simulink library "wind_gust_lib"  (R2015a)
settings: Solver=ode45  SolverMode=SingleTasking  StartTime=0.0  StopTime=10.0  RelTol=1e-3
undefined symbols (not defined in the file): a, b, Mq, Mw, Swg, Vto, Zw
libraries: simulink x1
settings Model: FPTRunName=Active  ModifiedByFormat=The MathWorks Inc.  CovSFcnEnable=off  ExtModeAutoUpdateStatusClock=off  Creator=The MathWorks Inc.  LastModifiedBy=The MathWorks Inc.
settings ConfigSet: ConfigType=Model
settings SolverCC: Priority=auto
settings DataIOCC: SignalLoggingSaveFormat=ModelDataLogs
settings OptimizationCC: BlockReduction=off  BooleanDataType=off  InlineParamsCompatibleMode=off  ExpressionDepthLimit=2147483647  ForceBlockIOInitOptimize=off  EvaledLifeSpan=1  SimCompilerOptimization=Off
settings DebuggingCC: SaveWithParameterizedLinksMsg=none  UnderspecifiedInitializationDetection=Classic  MergeDetectMultiDrivingBlocksExec=none  SignalResolutionControl=TryResolveAllWithWarning  FcnCallInpInsideContextMsg=EnableAllAsWarning  AllowSymbolicDim=off  StateNameClashWarn=warning  StrictBusMsg=Warning  SFMismatchInSimAndRtwBecauseOfMissingDataTypeDiag=warning
settings HardwareCC: TargetUnknown=on
settings RTWCC: EnableTagging=off  RTWCompilerOptimization=Off
settings CodeAppCC: ParameterTuningSideEffectCode=Output function  AllmanStyle=off
settings GRTTargetCC: CombineOutputUpdateFcns=off  EnableShiftOperators=off  PortableWordSizesTransition=off  GenerateErtSFunctionTransition=off  CreateSILPILBlockTransition=None  CodeProfilingSaveOptionsTransition=SummaryOnly  CodeExecutionProfilingTransition=off  CodeProfilingInstrumentationTransition=off  CodeExecutionProfileVariableTransition=executionProfile  GRTInterface=on

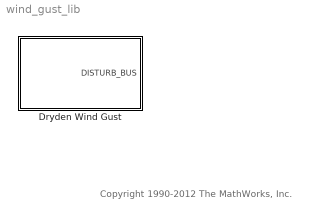
== system wind_gust_lib ==
  note: Copyright 1990-2012 The MathWorks, Inc.
  Dryden Wind Gust : Subsystem  IOType=none  Commented=off  StatePerturbationForJacobian=1.0e-05

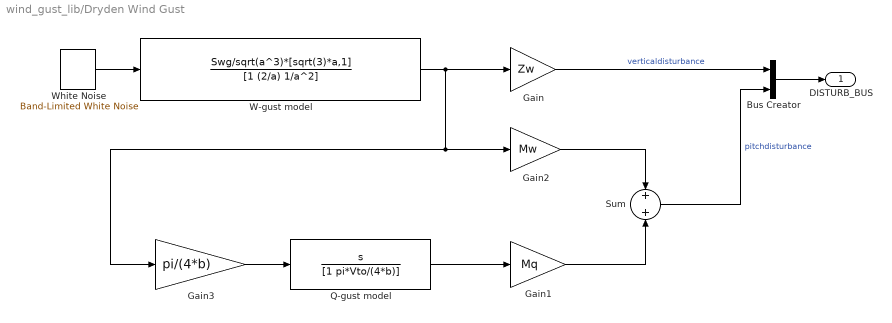
== system wind_gust_lib/Dryden Wind Gust ==
  Bus Creator : BusCreator  IOType=none  Commented=off  StatePerturbationForJacobian=1.0e-05  Inputs='verticaldisturbance','pitchdisturbance'  OutDataTypeStr=Bus: DISTURB_BUS
  Gain : Gain  IOType=none  Commented=off  StatePerturbationForJacobian=1.0e-05  Gain=Zw  SaturateOnIntegerOverflow=on  OutDataTypeStr=Inherit: Same as input  ParamDataTypeStr=Inherit: Same as input
  Gain1 : Gain  IOType=none  Commented=off  StatePerturbationForJacobian=1.0e-05  Gain=Mq  SaturateOnIntegerOverflow=on  OutDataTypeStr=Inherit: Same as input  ParamDataTypeStr=Inherit: Same as input
  Gain2 : Gain  IOType=none  Commented=off  StatePerturbationForJacobian=1.0e-05  Gain=Mw  SaturateOnIntegerOverflow=on  OutDataTypeStr=Inherit: Same as input  ParamDataTypeStr=Inherit: Same as input
  Gain3 : Gain  IOType=none  Commented=off  StatePerturbationForJacobian=1.0e-05  Gain=pi/(4*b)  SaturateOnIntegerOverflow=on  OutDataTypeStr=Inherit: Same as input  ParamDataTypeStr=Inherit: Same as input
  Q-gust model : TransferFcn  IOType=none  Commented=off  StatePerturbationForJacobian=1.0e-05  Numerator=[1 0]  Denominator=[1 pi*Vto/(4*b)]
  Sum : Sum  IOType=none  Commented=off  StatePerturbationForJacobian=1.0e-05  SaturateOnIntegerOverflow=on  InputSameDT=on  OutDataTypeStr=Inherit: Same as first input
  W-gust model : TransferFcn  IOType=none  Commented=off  StatePerturbationForJacobian=1.0e-05  Numerator=Swg/sqrt(a^3)*[sqrt(3)*a,1]  Denominator=[1 (2/a) 1/a^2]
  White Noise : simulink/Sources/Band-Limited White Noise  IOType=none  Commented=off  StatePerturbationForJacobian=1.0e-05  Cov=10  Ts=0.01  seed=23341
  DISTURB_BUS : Outport  IOType=none  Commented=off  StatePerturbationForJacobian=1.0e-05  OutDataTypeStr=Bus: DISTURB_BUS
  wires:
  Bus Creator/1 -> DISTURB_BUS/1
  Gain/1 -> Bus Creator/1  "verticaldisturbance"
  White Noise/1 -> W-gust model/1
  Gain3/1 -> Q-gust model/1
  Sum/1 -> Bus Creator/2  "pitchdisturbance"
  Gain2/1 -> Sum/1
  Gain1/1 -> Sum/2
  Q-gust model/1 -> Gain1/1
  W-gust model/1 -> Gain/1, Gain2/1, Gain3/1
